simulink model "power_PSS_modif"  (R2021b)
settings: Solver=ode23tb  StartTime=0.0  StopTime=20  MaxStep=1/60  RelTol=1e-3  EnableMultiTasking=on
undefined symbols (not defined in the file or in its folder): D1, Delta
libraries: spsThreePhaseFaultLib x11, spsGenericPowerSystemStabilizerLib x8, spsThreePhaseBreakerLib x6, spsThreePhaseParallelRLCLoadLib x6, spsLoadFlowBusLib x6, spsThreePhasePISectionLineLib x4, spsSynchronousMachinepuStandardLib x4, cstblocks x4, spsExcitationSystemLib x4, spsMultiBandPowerSystemStabilizerLib x4, spsSteamTurbineandGovernorLib x4, spsThreePhaseTransformerTwoWindingsLib x4
(part 1 of 2)
settings Model: FPTRunName=Active  Creator=The MathWorks, Inc.  LastModifiedBy=Pavel
settings SolverCC: ConsecutiveZCsStepRelTol=10*128*eps/2  AlgebraicLoopSolver=TrustRegion
settings DataIOCC: SaveFormat=Array  SaveOutput=off  SaveTime=off  ReturnWorkspaceOutputs=off  TimeSaveName=t  SignalLoggingName=sigsOut
settings OptimizationCC: BlockReduction=off  BooleanDataType=off  ExpressionDepthLimit=2147483647  InitFltsAndDblsToZero=on  LifeSpan=inf
settings DebuggingCC: UnderspecifiedInitializationDetection=Classic  MergeDetectMultiDrivingBlocksExec=none  SignalResolutionControl=TryResolveAllWithWarning  MultiTaskDSMMsg=warning  MultiTaskCondExecSysMsg=none  FcnCallInpInsideContextMsg=warning  UnconnectedInputMsg=none  UnconnectedOutputMsg=none  UnconnectedLineMsg=none  StateNameClashWarn=warning  SFUnexpectedBacktrackingDiag=warning  SFNoUnconditionalDefaultTransitionDiag=warning  SFExecutionAtInitializationDiag=none  SFMachineParentedDataDiag=warning  ArithmeticOperatorsInVariantConditions=warning
settings HardwareCC: ProdBitPerPointer=32  ProdBitPerSizeT=32  ProdBitPerPtrDiffT=32  ProdLargestAtomicFloat=None  ProdIntDivRoundTo=Undefined  ProdEndianess=Unspecified  ProdWordSize=32  ProdHWDeviceType=32-bit Generic  TargetUnknown=on
settings ModelReferenceCC: PropagateSignalLabelsOutOfModel=off
settings SFSimCC: SimUseLocalCustomCode=off  CustomCodeUndefinedFunction=UseInterfaceOnly
settings RTWCC: RTWUseLocalCustomCode=off
settings CodeAppCC: StateflowObjectComments=on
settings GRTTargetCC: TargetLangStandard=C89/C90 (ANSI)  CombineOutputUpdateFcns=off  GRTInterface=on
settings ConfigComp: CovMetricSettings=dw  CovSaveCumulativeToWorkspaceVar=on  CovSaveSingleToWorkspaceVar=on  CovExternalEMLEnable=off  CovSFcnEnable=off
settings SimscapeCC: SimscapeNormalizeSystem=off

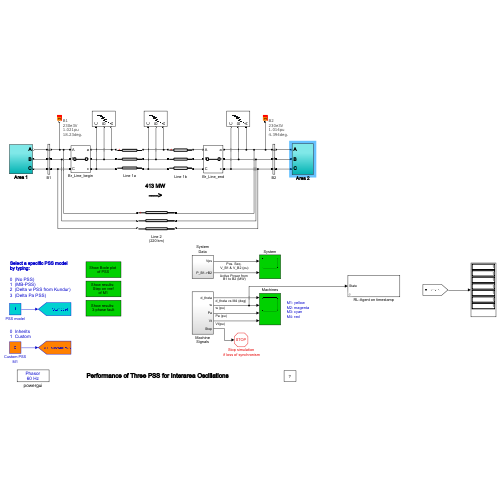
[thumbnail: Simulink's stored preview of the top-level diagram]
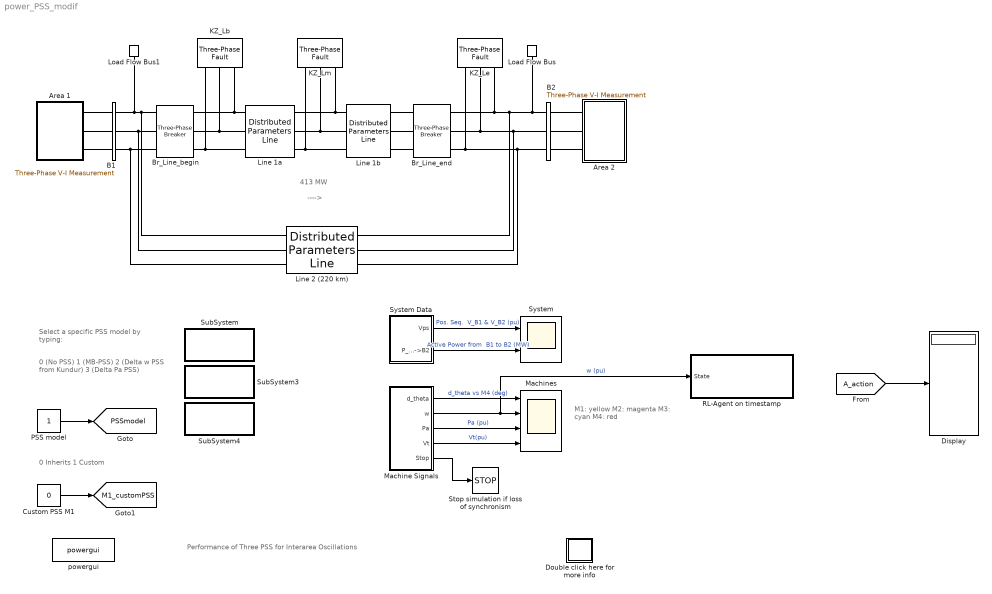
== system power_PSS_modif ==
  note: Performance of Three PSS for Interarea Oscillations
  note: M1: yellow
      | M2: magenta
      | M3: cyan
      | M4: red
  note: ---->
  note: 413 MW
  note: Select a specific PSS model
      | by typing:
  note: 0  (No PSS)
      | 1  (MB-PSS)
      | 2  (Delta w PSS from Kundur)
      | 3  (Delta Pa PSS)
  note: 0  Inherits
      | 1  Custom
  Area 1 : Subsystem
  Area 2 : Subsystem
  B1 : spsThreePhaseVIMeasurementLib/Three-Phase V-I Measurement  VoltageMeasurement=phase-to-ground  SetLabelV=on  LabelV=Vabc_B1  Vpu=off  VpuLL=off  CurrentMeasurement=yes  SetLabelI=on  LabelI=Iabc_B1  Ipu=off  Pbase=100e6  Vbase=500e3  OutputType=Complex  PhasorSimulation=on  PSBequivalent=0
  B2 : spsThreePhaseVIMeasurementLib/Three-Phase V-I Measurement  VoltageMeasurement=phase-to-ground  SetLabelV=on  LabelV=Vabc_B2  Vpu=off  VpuLL=off  CurrentMeasurement=yes  SetLabelI=on  LabelI=Iabc_B2  Ipu=off  Pbase=100e6  Vbase=500e3  OutputType=Complex  PhasorSimulation=on  PSBequivalent=0
  Br_Line_begin : spsThreePhaseBreakerLib/Three-Phase Breaker  InitialState=closed  SwitchA=on  SwitchB=on  SwitchC=on  SwitchTimes=[200]  External=off  BreakerResistance=0.001  SnubberResistance=inf  SnubberCapacitance=0  Measurements=None
      settings: AttributesFormatString=\n
  Br_Line_end : spsThreePhaseBreakerLib/Three-Phase Breaker  InitialState=closed  SwitchA=on  SwitchB=on  SwitchC=on  SwitchTimes=[200]  External=off  BreakerResistance=0.001  SnubberResistance=1e6  SnubberCapacitance=0  Measurements=None
      settings: AttributesFormatString=\n
  Custom PSS M1 : Constant  Value=0
  Display : Display
  Double click here for more info : Subsystem
      settings: OpenFcn=showdemo(bdroot(gcb))
      mask Display: disp('?')
  KZ_Lb : spsThreePhaseFaultLib/Three-Phase Fault  InitialStates=0  FaultA=off  FaultB=off  FaultC=off  GroundFault=on  SwitchTimes=[200]  External=off  SwitchStatus=NaN  FaultResistance=0.001  GroundResistance=0.001  SnubberResistance=1e6  SnubberCapacitance=inf  Measurements=None
  KZ_Le : spsThreePhaseFaultLib/Three-Phase Fault  InitialStates=0  FaultA=off  FaultB=off  FaultC=off  GroundFault=on  SwitchTimes=[200]  External=off  SwitchStatus=NaN  FaultResistance=0.001  GroundResistance=0.001  SnubberResistance=1e6  SnubberCapacitance=inf  Measurements=None
  KZ_Lm : spsThreePhaseFaultLib/Three-Phase Fault  InitialStates=0  FaultA=off  FaultB=off  FaultC=off  GroundFault=on  SwitchTimes=[200]  External=off  SwitchStatus=NaN  FaultResistance=0.001  GroundResistance=0.001  SnubberResistance=1e6  SnubberCapacitance=inf  Measurements=None
  Line 1a : spsDistributedParametersLineLib/Distributed Parameters Line  Phases=3  Length=110  Frequency=60  Resistance=[0.0529 1.61]  Inductance=[0.0014 0.0061]  Capacitance=[8.7749e-09 5.2489e-9]  x1=[1.03773522276635e-06 234865.712999227 234865.053199663;376.991118430775 376.991118430775 376.991118430775;-1.21492962029648 0.696371249684053 -0.874426885252841]  x2=[3.61832872068075e-07 234843.084420295 234843.00158467;376.991118430775 376.991118430775 376.991118430775;-0.99576107962275 0.574972704815849 -0.995825577248911]  x3=[1.73199030756503e-09 113.250290763104 113.254587804603;376.991118430775 376.991118430775 376.991118430775;0.426743142743769 0.12796103659155 -1.44291411331487]  x4=[2.20712280626888e-09 1062.45863712437 1062.45699915125;376.991118430775 376.991118430775 376.991118430775;-2.17151775162568 0.607648358429257 -0.963140711345587]  x5=0.000622431770558027  V1=ones(3,3)  V2=ones(3,3)  I1=ones(3,3)  I2=ones(3,3)  nHarmo=1  Measurements=None  Decoupling=off  VsMag0=0  VrMag0=0  VsAngle0=0  VrAngle0=0  IsMag0=0  IrMag0=0  IsAngle0=0  IrAngle0=0
      settings: AttributesFormatString=\n  SourceProductBaseCode=PS
  Line 1b : spsDistributedParametersLineLib/Distributed Parameters Line  Phases=3  Length=110  Frequency=60  Resistance=[0.0529 1.61]  Inductance=[0.0014 0.0061]  Capacitance=[8.7749e-09 5.2489e-9]  x1=[3.61827603793127e-07 234843.084420295 234843.00158467;376.991118430775 376.991118430775 376.991118430775;-0.995774949247956 0.574972704815849 -0.995825577248911]  x2=[3.91159002907788e-07 233276.177129905 233276.6633314;376.991118430775 376.991118430775 376.991118430775;1.48599709564018 0.454941358463387 -1.11585647609775]  x3=[2.05241143482151e-09 107.229638862451 107.234251771631;376.991118430775 376.991118430775 376.991118430775;0.699241722974643 0.245334104052737 -1.32554535066755]  x4=[1.87375449005804e-09 1055.26028297532 1055.25866903581;376.991118430775 376.991118430775 376.991118430775;-2.39378343032615 0.462097686461629 -1.10869145435477]  x5=0.000622431770558027  V1=ones(3,3)  V2=ones(3,3)  I1=ones(3,3)  I2=ones(3,3)  nHarmo=1  Measurements=None  Decoupling=off  VsMag0=0  VrMag0=0  VsAngle0=0  VrAngle0=0  IsMag0=0  IrMag0=0  IsAngle0=0  IrAngle0=0
      settings: AttributesFormatString=\n  SourceProductBaseCode=PS
  Line 2 (220 km) : spsDistributedParametersLineLib/Distributed Parameters Line  Phases=3  Length=220  Frequency=60  Resistance=[0.0001*529 1.61]  Inductance=[0.001*529/(377) 0.0061]  Capacitance=[0.00175/529/(377) 5.2489e-9]  x1=[1.03587220395795e-06 234866.202959166 234865.543159038;376.991118430775 376.991118430775 376.991118430775;-1.45669181718141 0.550693672846279 -1.02010446204846]  x2=[3.84671171209545e-07 233275.696082472 233276.182286874;376.991118430775 376.991118430775 376.991118430775;1.25538564201445 0.309263487558995 -1.26153434704163]  x3=[1.59106685653725e-09 111.016553993005 111.020863873188;376.991118430775 376.991118430775 376.991118430775;0.203367965270843 -0.0239956419974053 -1.59487136078097]  x4=[1.73228997364306e-09 1043.99344327446 1043.99184261649;376.991118430775 376.991118430775 376.991118430775;-2.6313512786114 0.316034427449977 -1.25475470203141]  x5=0.00124486354111605  V1=ones(3,3)  V2=ones(3,3)  I1=ones(3,3)  I2=ones(3,3)  nHarmo=1  Measurements=None  Decoupling=off  VsMag0=0  VrMag0=0  VsAngle0=0  VrAngle0=0  IsMag0=0  IrMag0=0  IsAngle0=0  IrAngle0=0
      settings: AttributesFormatString=\n  SourceProductBaseCode=PS
  Load Flow Bus : spsLoadFlowBusLib/Load Flow Bus  LConnTagsString=a  Phases=single  Connectors=on one side  ID=B2  Vbase=230e3  Vref=1  Vangle=0  VLF=1.014  VLFb=1  VLFc=1  angleLF=4.394  angleLFb=0  angleLFc=0
      settings: AttributesFormatString=%<ID>\n%<Vbase>V\n%<VLF>pu\n%<angleLF>deg.  SourceProductBaseCode=PS
  Load Flow Bus1 : spsLoadFlowBusLib/Load Flow Bus  LConnTagsString=a  Phases=single  Connectors=on one side  ID=B1  Vbase=230e3  Vref=1  Vangle=0  VLF=1.021  VLFb=1  VLFc=1  angleLF=18.23  angleLFb=0  angleLFc=0
      settings: AttributesFormatString=%<ID>\n%<Vbase>V\n%<VLF>pu\n%<angleLF>deg.  SourceProductBaseCode=PS
  Machine Signals : Subsystem
  Machines : Scope  NumInputPorts=4
  PSS model : Constant
  RL-Agent on timestamp : Subsystem  mask{period=1, swi_threshlod=1.1, initPSSParams=[1 1 1 1 1 1 1]}
      mask prompts: period "Period (s)"; swi_threshlod "Switch threshold (s)"; initPSSParams "Initial PSS parameters"
  Stop simulation if loss of synchronism : Stop
  SubSystem : Subsystem
      settings: OpenFcn=openfig('psbPSSbode.fig');
      mask Display: disp('Show Bode plot \nof PSS')
  SubSystem3 : Subsystem
      settings: OpenFcn=openfig('psbPSSstep.fig');
      mask Display: disp('Show results: \nStep on vref\nof M1')
  SubSystem4 : Subsystem
      settings: OpenFcn=openfig('psbPSSfault.fig');
      mask Display: disp('Show results: \n3-phase fault')
  System : Scope  NumInputPorts=2
  System Data : Subsystem
  powergui : spspowerguiLib/powergui  Priority=2  SimulationMode=Phasor  SampleTime=0  frequency=60  Iterations=50  frequencyindice=60  Pbase=100e6  ErrMax=0.0001  UnitsV=kV  UnitsW=MW  buscounter=0  FunctionMessages=off  echomessages=off  EnableUseOfTLC=off  CurrentSourceSwitches=off  DisableSnubberDevices=off  DisableRonSwitches=off  DisableVfSwitches=off  DisplayEquations=off  AutomaticDiscreteSolvers=off  SolverType=Tustin  Interpol=off  ExternalGateDelay=off  methode=off  Ts=0  x0status=blocks  SPID=off  SwTol=0  HookPort=off  NonlinearTolerance=1e-4  nMaxIteration=100  ContinueOnMaxIteration=off  RestoreLinks=warning  ResistiveCurrentMeasurement=off  Frange=logspace(0,3,50)  Ylog=off  Xlog=off  ShowGrid=off  save=off  variable=ZData  structure=0  ZoomFFT=on  StartTime=0.0  cycles=1  DisplayStyle=1  fundamental=60  FreqAxis=off  MaxFrequency=1000  frequencyindicesteady=1  RmsSteady=1  display=off
  tag scope: M1_customPSS=global, PSSmodel=global
  wires:
  Machine Signals/1(d_theta) -> Machines/1  "d_theta vs M4 (deg)"
  Machine Signals/2(w) -> RL-Agent on timestamp/1(State), Machines/2  "w (pu)"
  Machine Signals/3(Pa) -> Machines/3  "Pa (pu)"
  Machine Signals/4(Vt) -> Machines/4  "Vt(pu)"
  Machine Signals/5(Stop) -> Stop simulation if loss of synchronism/1
  System Data/1(Vps) -> System/1  "Pos. Seq.  V_B1 & V_B2 (pu)"
  System Data/2(P_B1->B2) -> System/2  "Active Power from  B1 to B2 (MW)"
  PSS model/1 -> [PSSmodel]
  [A_action] -> Display/1
  Custom PSS M1/1 -> [M1_customPSS]
  connections:
  Br_Line_begin/RConn1 -- KZ_Lb/LConn1 -- Line 1a/LConn1
  Br_Line_begin/RConn2 -- KZ_Lb/LConn2 -- Line 1a/LConn2
  Br_Line_begin/RConn3 -- KZ_Lb/LConn3 -- Line 1a/LConn3
  Line 1b/LConn1 -- KZ_Lm/LConn1 -- Line 1a/RConn1
  Line 1b/LConn2 -- KZ_Lm/LConn2 -- Line 1a/RConn2
  Line 1a/RConn3 -- KZ_Lm/LConn3 -- Line 1b/LConn3
  Line 1b/RConn1 -- Br_Line_end/LConn1
  Line 1b/RConn2 -- Br_Line_end/LConn2
  Line 1b/RConn3 -- Br_Line_end/LConn3
  Area 1/RConn2 -- B1/LConn2
  Area 1/RConn1 -- B1/LConn1
  Area 1/RConn3 -- B1/LConn3
  B1/RConn2 -- Br_Line_begin/LConn2 -- Line 2 (220 km)/LConn2
  B1/RConn1 -- Br_Line_begin/LConn1 -- Line 2 (220 km)/LConn1 -- Load Flow Bus1/LConn1
  B1/RConn3 -- Br_Line_begin/LConn3 -- Line 2 (220 km)/LConn3
  B2/RConn2 -- Area 2/LConn2
  B2/RConn1 -- Area 2/LConn1
  B2/RConn3 -- Area 2/LConn3
  B2/LConn2 -- KZ_Le/LConn2 -- Br_Line_end/RConn2 -- Line 2 (220 km)/RConn2
  B2/LConn1 -- KZ_Le/LConn1 -- Br_Line_end/RConn1 -- Line 2 (220 km)/RConn1 -- Load Flow Bus/LConn1
  B2/LConn3 -- KZ_Le/LConn3 -- Br_Line_end/RConn3 -- Line 2 (220 km)/RConn3

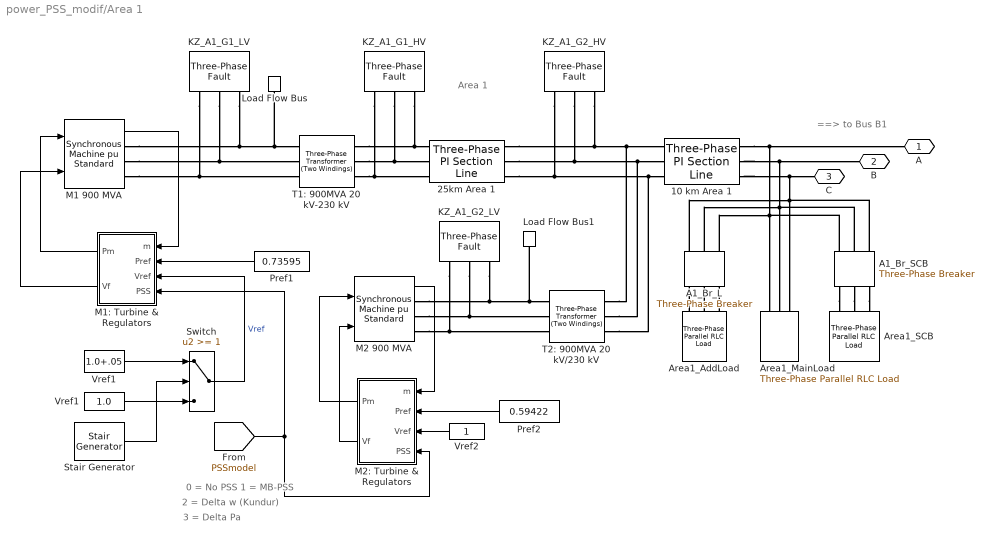
== system power_PSS_modif/Area 1 ==
  note: Area 1
  note: ==> to Bus B1
  note: 0 = No PSS
      | 1 = MB-PSS
  note: 3 = Delta Pa
  note: 2 = Delta w (Kundur)
  10 km Area 1 : spsThreePhasePISectionLineLib/Three-Phase PI Section Line  LConnTagsString=a|b|c  RConnTagsString=A|B|C  Length=10  Frequency=60  Resistances=[0.0529 1.61]  Inductances=[0.0014 0.0061]  Capacitances=[8.7749e-09 5.2489e-9]
  25km Area 1 : spsThreePhasePISectionLineLib/Three-Phase PI Section Line  LConnTagsString=a|b|c  RConnTagsString=A|B|C  Length=25  Frequency=60  Resistances=[0.0529 1.61]  Inductances=[0.0014 0.0061]  Capacitances=[8.7749e-09 5.2489e-9]
  A1_Br_L : spsThreePhaseBreakerLib/Three-Phase Breaker  InitialState=open  SwitchA=on  SwitchB=on  SwitchC=on  SwitchTimes=[200]  External=off  BreakerResistance=0.001  SnubberResistance=inf  SnubberCapacitance=0  Measurements=None
      settings: AttributesFormatString=\n
  A1_Br_SCB : spsThreePhaseBreakerLib/Three-Phase Breaker  InitialState=closed  SwitchA=on  SwitchB=on  SwitchC=on  SwitchTimes=[200]  External=off  BreakerResistance=0.001  SnubberResistance=inf  SnubberCapacitance=0  Measurements=None
      settings: AttributesFormatString=\n
  Area1_AddLoad : spsThreePhaseParallelRLCLoadLib/Three-Phase Parallel RLC Load  LConnTagsString=A|B|C  Configuration=Y (grounded)  NominalVoltage=230e3  Vabc=[1e3 1e3 1e3]  Vabcp=[1e3 1e3 1e3]  NominalFrequency=60  UnbalancedPower=off  ActivePower=1  InductivePower=0  CapacitivePower=0  Pabc=[10e3 9e3 11e3]  QLabc=[100 90 110]  QCabc=[100 90 110]  Pabcp=[10e3 9e3 11e3]  QLabcp=[100 90 110]  QCabcp=[100 90 110]  Measurements=None  LoadType=constant Z
  Area1_MainLoad : spsThreePhaseParallelRLCLoadLib/Three-Phase Parallel RLC Load  LConnTagsString=A|B|C  Configuration=Y (grounded)  NominalVoltage=230e3  Vabc=[1e3 1e3 1e3]  Vabcp=[1e3 1e3 1e3]  NominalFrequency=60  UnbalancedPower=off  ActivePower=900000000  InductivePower=0  CapacitivePower=100000000  Pabc=[10e3 9e3 11e3]  QLabc=[100 90 110]  QCabc=[100 90 110]  Pabcp=[10e3 9e3 11e3]  QLabcp=[100 90 110]  QCabcp=[100 90 110]  Measurements=None  LoadType=constant Z
  Area1_SCB : spsThreePhaseParallelRLCLoadLib/Three-Phase Parallel RLC Load  LConnTagsString=A|B|C  Configuration=Y (grounded)  NominalVoltage=230e3  Vabc=[1e3 1e3 1e3]  Vabcp=[1e3 1e3 1e3]  NominalFrequency=60  UnbalancedPower=off  ActivePower=0  InductivePower=0  CapacitivePower=200000000  Pabc=[10e3 9e3 11e3]  QLabc=[100 90 110]  QCabc=[100 90 110]  Pabcp=[10e3 9e3 11e3]  QLabcp=[100 90 110]  QCabcp=[100 90 110]  Measurements=None  LoadType=constant Z
  KZ_A1_G1_HV : spsThreePhaseFaultLib/Three-Phase Fault  InitialStates=0  FaultA=off  FaultB=off  FaultC=off  GroundFault=on  SwitchTimes=[200]  External=off  SwitchStatus=NaN  FaultResistance=0.001  GroundResistance=0.001  SnubberResistance=1e6  SnubberCapacitance=inf  Measurements=None
  KZ_A1_G1_LV : spsThreePhaseFaultLib/Three-Phase Fault  InitialStates=0  FaultA=off  FaultB=off  FaultC=off  GroundFault=on  SwitchTimes=[200]  External=off  SwitchStatus=NaN  FaultResistance=0.001  GroundResistance=0.001  SnubberResistance=1e6  SnubberCapacitance=inf  Measurements=None
  KZ_A1_G2_HV : spsThreePhaseFaultLib/Three-Phase Fault  InitialStates=0  FaultA=on  FaultB=on  FaultC=on  GroundFault=on  SwitchTimes=[200]  External=off  SwitchStatus=NaN  FaultResistance=0.001  GroundResistance=0.001  SnubberResistance=1e6  SnubberCapacitance=inf  Measurements=None
  KZ_A1_G2_LV : spsThreePhaseFaultLib/Three-Phase Fault  InitialStates=0  FaultA=off  FaultB=off  FaultC=off  GroundFault=on  SwitchTimes=[200]  External=off  SwitchStatus=NaN  FaultResistance=0.001  GroundResistance=0.001  SnubberResistance=1e6  SnubberCapacitance=inf  Measurements=None
  Load Flow Bus : spsLoadFlowBusLib/Load Flow Bus  LConnTagsString=a  Phases=single  Connectors=on one side  ID=M1_Area1  Vbase=20e3  Vref=1  Vangle=0  VLF=1  VLFb=1  VLFc=1  angleLF=10.73  angleLFb=0  angleLFc=0
      settings: AttributesFormatString=%<ID>\n%<Vbase>V\n%<VLF>pu\n%<angleLF>deg.  SourceProductBaseCode=PS
  Load Flow Bus1 : spsLoadFlowBusLib/Load Flow Bus  LConnTagsString=a  Phases=single  Connectors=on one side  ID=M2_Area1  Vbase=20e3  Vref=1  Vangle=0  VLF=1  VLFb=1  VLFc=1  angleLF=0  angleLFb=0  angleLFc=0
      settings: AttributesFormatString=%<ID>\n%<Vbase>V\n%<VLF>pu\n%<angleLF>deg.  SourceProductBaseCode=PS
  M1 900 MVA : spsSynchronousMachinepuStandardLib/Synchronous Machine pu Standard  PresetModel=No  MechanicalLoad=Mechanical power Pm  ShowDetailedParameters=on  RotorType=Round  Units=per unit standard parameters  MeasurementBus=off  NominalParameters="[900E6  20000   60 ]"  Reactances1=[1.8 .3 .25 1.7 .55 .25 .2]  Reactances2=[ 1.305, 0.296, 0.252, 0.474, 0.243, 0.18 ]  dAxisTimeConstants=Open-circuit  qAxisTimeConstants=Open-circuit  TimeConstants1=[]  TimeConstants2=[8 .03 .4 .05]  TimeConstants3=[]  TimeConstants4=[]  TimeConstants5=[ 1.01, 0.053, 0.1 ]  TimeConstants6=[]  TimeConstants7=[]  TimeConstants8=[]  StatorResistance=0.0025  Mechanical=[ 6.5 0 4]  PolePairs=4  InitialConditions=[0 -29.8925 0.737138 0.737138 0.737138 7.47241 -112.528 127.472 1.70671]  SetSaturation=off  Saturation=[0.6404,0.7127,0.8441,0.9214,0.9956,1.082,1.19,1.316,1.457;0.7,0.7698,0.8872,0.9466,0.9969,1.046,1.1,1.151,1.201]  LoadFlowParameters=[1 700000000 0 0 0]  TsPowergui=0  TsBlock=-1  IterativeModel=Trapezoidal non iterative  IterativeDiscreteModel=Trapezoidal non iterative  BusType=PV  Pref=662353696.8626  Qref=0  Qmin=-Inf  Qmax=Inf  PLF=0  QLF=0
      settings: SourceProductBaseCode=PS
  M1: Turbine & Regulators : Subsystem
  M2 900 MVA : spsSynchronousMachinepuStandardLib/Synchronous Machine pu Standard  PresetModel=No  MechanicalLoad=Mechanical power Pm  ShowDetailedParameters=on  RotorType=Round  Units=per unit standard parameters  MeasurementBus=off  NominalParameters="[900E6  20000   60 ]"  Reactances1=[1.8 .3 .25 1.7 .55 .25 .2]  Reactances2=[ 1.305, 0.296, 0.252, 0.474, 0.243, 0.18 ]  dAxisTimeConstants=Open-circuit  qAxisTimeConstants=Open-circuit  TimeConstants1=[]  TimeConstants2=[8 .03 .4 .05]  TimeConstants3=[]  TimeConstants4=[]  TimeConstants5=[ 1.01, 0.053, 0.1 ]  TimeConstants6=[]  TimeConstants7=[]  TimeConstants8=[]  StatorResistance=0.0025  Mechanical=[ 6.5 0 4]  PolePairs=4  InitialConditions=[0 -44.1681 0.594337 0.594337 0.594337 1.14574 -118.854 121.146 1.45014]  SetSaturation=off  Saturation=[0.6404,0.7127,0.8441,0.9214,0.9956,1.082,1.19,1.316,1.457;0.7,0.7698,0.8872,0.9466,0.9969,1.046,1.1,1.151,1.201]  LoadFlowParameters=[2 700000000 0 0 0]  TsPowergui=0  TsBlock=-1  IterativeModel=Trapezoidal non iterative  IterativeDiscreteModel=Trapezoidal non iterative  BusType=swing  Pref=754208614.3715  Qref=0  Qmin=-Inf  Qmax=Inf  PLF=0  QLF=0
      settings: SourceProductBaseCode=PS
  M2: Turbine & Regulators : Subsystem
  Pref1 : Constant  Value=0.73595
  Pref2 : Constant  Value=0.59422
  Stair Generator : spsStairGeneratorLib/Stair Generator  t=[0 1 1.2]*100  e=[0 1 0 ]  Ts=0
  Switch : Switch  Threshold=1  InputSameDT=on
  T1: 900MVA 20 kV-230 kV : spsThreePhaseTransformerTwoWindingsLib/Three-Phase Transformer (Two Windings)  Winding1Connection=Delta (D1)  Winding2Connection=Yg  CoreType=Three single-phase transformers  SetSaturation=off  Hysteresis=off  DataFile='hysteresis'  SetInitialFlux=off  Measurements=None  UNITS=pu  NominalPower="[ 900e6   60 ]"  Winding1="[ 20e3  1e-6   0  ]"  Winding2="[ 230e3  1e-6   0.15 ]"  Rm=500  Lm=500  L0=0.5  Saturation="[ 0,0  ;  0.005,1.2  ;  1.0,1.4 ]"  InitialFluxes=[ 0.8 , -0.8 , 0.7 ]  BreakLoop=off  DiscreteSolver=Trapezoidal iterative  DataType=off  TransfoNumber=0
  T2: 900MVA 20 kV/230 kV : spsThreePhaseTransformerTwoWindingsLib/Three-Phase Transformer (Two Windings)  Winding1Connection=Delta (D1)  Winding2Connection=Yg  CoreType=Three single-phase transformers  SetSaturation=off  Hysteresis=off  DataFile='hysteresis'  SetInitialFlux=off  Measurements=None  UNITS=pu  NominalPower=[ 900e6 60 ]  Winding1="[ 20e3 1e-6  0.0]"  Winding2=[ 230e3 1e-6 0.15]  Rm=500  Lm=500  L0=0.5  Saturation="[ 0,0  ;  0.005,1.2  ;  1.0,1.4 ]"  InitialFluxes=[ 0.8 , -0.8 , 0.7 ]  BreakLoop=off  DiscreteSolver=Trapezoidal iterative  DataType=off  TransfoNumber=0
  Vref1 : Constant  Value=1.0
  "Vref1 " : Constant  Value=1.0+.05
  Vref2 : Constant
  " A" : PMIOPort  Side=Right
  " B" : PMIOPort  Port=2  Side=Right
  " C" : PMIOPort  Port=3  Side=Right
  wires:
  Pref1/1 -> M1: Turbine & Regulators/2(Pref)
  Switch/1 -> M1: Turbine & Regulators/3(Vref)  "Vref"
  Stair Generator/1 -> Switch/2
  [PSSmodel] -> M1: Turbine & Regulators/4(PSS), M2: Turbine & Regulators/4(PSS)
  Pref2/1 -> M2: Turbine & Regulators/2(Pref)
  Vref2/1 -> M2: Turbine & Regulators/3(Vref)
  Vref1/1 -> Switch/3
  "Vref1 "/1 -> Switch/1
  M2 900 MVA/1 -> M2: Turbine & Regulators/1(m)
  M2: Turbine & Regulators/1(Pm) -> M2 900 MVA/1
  M2: Turbine & Regulators/2(Vf) -> M2 900 MVA/2
  M1: Turbine & Regulators/1(Pm) -> M1 900 MVA/1
  M1: Turbine & Regulators/2(Vf) -> M1 900 MVA/2
  M1 900 MVA/1 -> M1: Turbine & Regulators/1(m)
  connections:
  T1: 900MVA 20 kV-230 kV/RConn1 -- KZ_A1_G1_HV/LConn1 -- 25km Area 1/LConn1
  T1: 900MVA 20 kV-230 kV/RConn2 -- KZ_A1_G1_HV/LConn2 -- 25km Area 1/LConn2
  M2 900 MVA/RConn1 -- KZ_A1_G2_LV/LConn1 -- T2: 900MVA 20 kV/230 kV/LConn1 -- Load Flow Bus1/LConn1
  M2 900 MVA/RConn2 -- KZ_A1_G2_LV/LConn2 -- T2: 900MVA 20 kV/230 kV/LConn2
  M2 900 MVA/RConn3 -- KZ_A1_G2_LV/LConn3 -- T2: 900MVA 20 kV/230 kV/LConn3
  T1: 900MVA 20 kV-230 kV/RConn3 -- KZ_A1_G1_HV/LConn3 -- 25km Area 1/LConn3
  10 km Area 1/RConn1 -- " A"/RConn1 -- A1_Br_L/RConn3 -- A1_Br_SCB/RConn1 -- Area1_MainLoad/LConn1
  10 km Area 1/RConn2 -- " B"/RConn1 -- A1_Br_L/RConn2 -- A1_Br_SCB/RConn2 -- Area1_MainLoad/LConn2
  10 km Area 1/RConn3 -- " C"/RConn1 -- A1_Br_L/RConn1 -- A1_Br_SCB/RConn3 -- Area1_MainLoad/LConn3
  M1 900 MVA/RConn1 -- KZ_A1_G1_LV/LConn1 -- T1: 900MVA 20 kV-230 kV/LConn1 -- Load Flow Bus/LConn1
  M1 900 MVA/RConn2 -- KZ_A1_G1_LV/LConn2 -- T1: 900MVA 20 kV-230 kV/LConn2
  M1 900 MVA/RConn3 -- KZ_A1_G1_LV/LConn3 -- T1: 900MVA 20 kV-230 kV/LConn3
  25km Area 1/RConn2 -- KZ_A1_G2_HV/LConn2 -- T2: 900MVA 20 kV/230 kV/RConn2 -- 10 km Area 1/LConn2
  25km Area 1/RConn1 -- KZ_A1_G2_HV/LConn1 -- T2: 900MVA 20 kV/230 kV/RConn1 -- 10 km Area 1/LConn1
  25km Area 1/RConn3 -- KZ_A1_G2_HV/LConn3 -- T2: 900MVA 20 kV/230 kV/RConn3 -- 10 km Area 1/LConn3
  A1_Br_SCB/LConn1 -- Area1_SCB/LConn1
  A1_Br_SCB/LConn2 -- Area1_SCB/LConn2
  A1_Br_SCB/LConn3 -- Area1_SCB/LConn3
  Area1_AddLoad/LConn1 -- A1_Br_L/LConn1
  Area1_AddLoad/LConn3 -- A1_Br_L/LConn3
  Area1_AddLoad/LConn2 -- A1_Br_L/LConn2

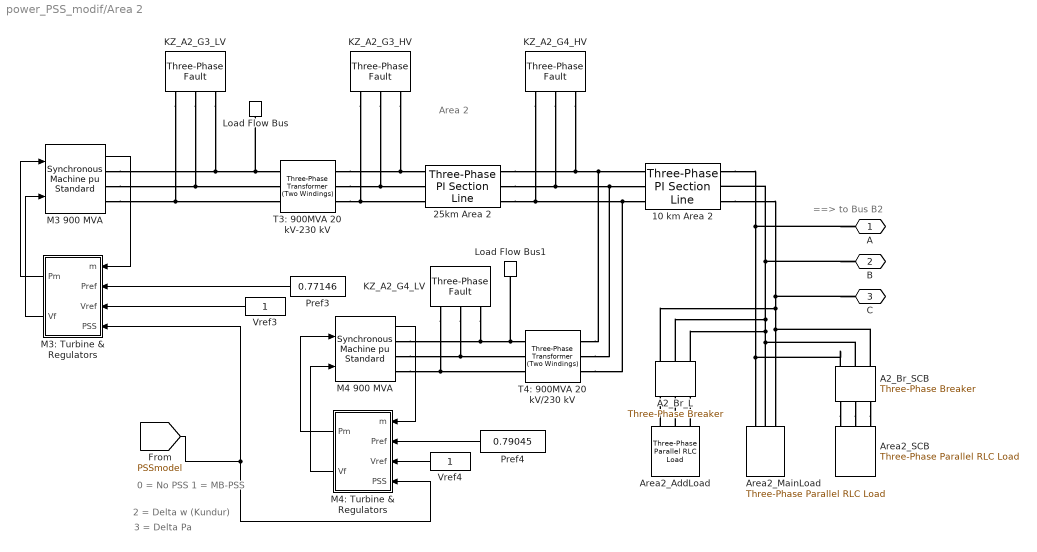
== system power_PSS_modif/Area 2 ==
  note: 2 = Delta w (Kundur)
  note: 3 = Delta Pa
  note: 0 = No PSS
      | 1 = MB-PSS
  note: ==> to Bus B2
  note: Area 2
  10 km Area 2 : spsThreePhasePISectionLineLib/Three-Phase PI Section Line  LConnTagsString=a|b|c  RConnTagsString=A|B|C  Length=10  Frequency=60  Resistances=[0.0529 1.61]  Inductances=[0.0014 0.0061]  Capacitances=[8.7749e-09 5.2489e-9]
  25km Area 2 : spsThreePhasePISectionLineLib/Three-Phase PI Section Line  LConnTagsString=a|b|c  RConnTagsString=A|B|C  Length=25  Frequency=60  Resistances=[0.0529 1.61]  Inductances=[0.0014 0.0061]  Capacitances=[8.7749e-09 5.2489e-9]
  A2_Br_L : spsThreePhaseBreakerLib/Three-Phase Breaker  InitialState=open  SwitchA=on  SwitchB=on  SwitchC=on  SwitchTimes=[200]  External=off  BreakerResistance=0.001  SnubberResistance=inf  SnubberCapacitance=0  Measurements=None
      settings: AttributesFormatString=\n
  A2_Br_SCB : spsThreePhaseBreakerLib/Three-Phase Breaker  InitialState=closed  SwitchA=on  SwitchB=on  SwitchC=on  SwitchTimes=[200]  External=off  BreakerResistance=0.001  SnubberResistance=inf  SnubberCapacitance=0  Measurements=None
      settings: AttributesFormatString=\n
  Area2_AddLoad : spsThreePhaseParallelRLCLoadLib/Three-Phase Parallel RLC Load  LConnTagsString=A|B|C  Configuration=Y (grounded)  NominalVoltage=230e3  Vabc=[1e3 1e3 1e3]  Vabcp=[1e3 1e3 1e3]  NominalFrequency=60  UnbalancedPower=off  ActivePower=200  InductivePower=0  CapacitivePower=1  Pabc=[10e3 9e3 11e3]  QLabc=[100 90 110]  QCabc=[100 90 110]  Pabcp=[10e3 9e3 11e3]  QLabcp=[100 90 110]  QCabcp=[100 90 110]  Measurements=None  LoadType=constant Z
  Area2_MainLoad : spsThreePhaseParallelRLCLoadLib/Three-Phase Parallel RLC Load  LConnTagsString=A|B|C  Configuration=Y (grounded)  NominalVoltage=230e3  Vabc=[1e3 1e3 1e3]  Vabcp=[1e3 1e3 1e3]  NominalFrequency=60  UnbalancedPower=off  ActivePower=1550000000  InductivePower=0  CapacitivePower=19684279.1507  Pabc=[10e3 9e3 11e3]  QLabc=[100 90 110]  QCabc=[100 90 110]  Pabcp=[10e3 9e3 11e3]  QLabcp=[100 90 110]  QCabcp=[100 90 110]  Measurements=None  LoadType=constant Z
  Area2_SCB : spsThreePhaseParallelRLCLoadLib/Three-Phase Parallel RLC Load  LConnTagsString=A|B|C  Configuration=Y (grounded)  NominalVoltage=230e3  Vabc=[1e3 1e3 1e3]  Vabcp=[1e3 1e3 1e3]  NominalFrequency=60  UnbalancedPower=off  ActivePower=0  InductivePower=0  CapacitivePower=350000000  Pabc=[10e3 9e3 11e3]  QLabc=[100 90 110]  QCabc=[100 90 110]  Pabcp=[10e3 9e3 11e3]  QLabcp=[100 90 110]  QCabcp=[100 90 110]  Measurements=None  LoadType=constant Z
  KZ_A2_G3_HV : spsThreePhaseFaultLib/Three-Phase Fault  InitialStates=0  FaultA=off  FaultB=off  FaultC=off  GroundFault=on  SwitchTimes=[200]  External=off  SwitchStatus=NaN  FaultResistance=0.001  GroundResistance=0.001  SnubberResistance=1e6  SnubberCapacitance=inf  Measurements=None
  KZ_A2_G3_LV : spsThreePhaseFaultLib/Three-Phase Fault  InitialStates=0  FaultA=off  FaultB=off  FaultC=off  GroundFault=on  SwitchTimes=[200]  External=off  SwitchStatus=NaN  FaultResistance=0.001  GroundResistance=0.001  SnubberResistance=1e6  SnubberCapacitance=inf  Measurements=None
  KZ_A2_G4_HV : spsThreePhaseFaultLib/Three-Phase Fault  InitialStates=0  FaultA=off  FaultB=off  FaultC=off  GroundFault=on  SwitchTimes=[200]  External=off  SwitchStatus=NaN  FaultResistance=0.001  GroundResistance=0.001  SnubberResistance=1e6  SnubberCapacitance=inf  Measurements=None
  KZ_A2_G4_LV : spsThreePhaseFaultLib/Three-Phase Fault  InitialStates=0  FaultA=off  FaultB=off  FaultC=off  GroundFault=on  SwitchTimes=[200]  External=off  SwitchStatus=NaN  FaultResistance=0.001  GroundResistance=0.001  SnubberResistance=1e6  SnubberCapacitance=inf  Measurements=None
  Load Flow Bus : spsLoadFlowBusLib/Load Flow Bus  LConnTagsString=a  Phases=single  Connectors=on one side  ID=M3_Area2  Vbase=20e3  Vref=1  Vangle=0  VLF=1  VLFb=1  VLFc=1  angleLF=-0.9983  angleLFb=0  angleLFc=0
      settings: AttributesFormatString=%<ID>\n%<Vbase>V\n%<VLF>pu\n%<angleLF>deg.  SourceProductBaseCode=PS
  Load Flow Bus1 : spsLoadFlowBusLib/Load Flow Bus  LConnTagsString=a  Phases=single  Connectors=on one side  ID=M4_Area2  Vbase=20e3  Vref=1  Vangle=0  VLF=1  VLFb=1  VLFc=1  angleLF=-10.86  angleLFb=0  angleLFc=0
      settings: AttributesFormatString=%<ID>\n%<Vbase>V\n%<VLF>pu\n%<angleLF>deg.  SourceProductBaseCode=PS
  M3 900 MVA : spsSynchronousMachinepuStandardLib/Synchronous Machine pu Standard  PresetModel=No  MechanicalLoad=Mechanical power Pm  ShowDetailedParameters=on  RotorType=Round  Units=per unit standard parameters  MeasurementBus=off  NominalParameters="[900E6  20000   60 ]"  Reactances1=[1.8 .3 .25 1.7 .55 .25 .2]  Reactances2=[ 1.305, 0.296, 0.252, 0.474, 0.243, 0.18 ]  dAxisTimeConstants=Open-circuit  qAxisTimeConstants=Open-circuit  TimeConstants1=[]  TimeConstants2=[8 .03 .4 .05]  TimeConstants3=[]  TimeConstants4=[]  TimeConstants5=[ 1.01, 0.053, 0.1 ]  TimeConstants6=[]  TimeConstants7=[]  TimeConstants8=[]  StatorResistance=0.0025  Mechanical=[ 6.175 0 4]  PolePairs=4  InitialConditions=[0 -41.3376 0.77425 0.77425 0.77425 -5.86613 -125.866 114.134 1.78343]  SetSaturation=off  Saturation=[0.6404,0.7127,0.8441,0.9214,0.9956,1.082,1.19,1.316,1.457;0.7,0.7698,0.8872,0.9466,0.9969,1.046,1.1,1.151,1.201]  LoadFlowParameters=[1 719000000 0 0 0]  TsPowergui=0  TsBlock=-1  IterativeModel=Trapezoidal non iterative  IterativeDiscreteModel=Trapezoidal non iterative  BusType=PV  Pref=694311768.0691  Qref=0  Qmin=-Inf  Qmax=Inf  PLF=0  QLF=0
      settings: SourceProductBaseCode=PS
  M3: Turbine & Regulators : Subsystem
  M4 900 MVA : spsSynchronousMachinepuStandardLib/Synchronous Machine pu Standard  PresetModel=No  MechanicalLoad=Mechanical power Pm  ShowDetailedParameters=on  RotorType=Round  Units=per unit standard parameters  MeasurementBus=off  NominalParameters="[900E6  20000   60 ]"  Reactances1=[1.8 .3 .25 1.7 .55 .25 .2]  Reactances2=[ 1.305, 0.296, 0.252, 0.474, 0.243, 0.18 ]  dAxisTimeConstants=Open-circuit  qAxisTimeConstants=Open-circuit  TimeConstants1=[]  TimeConstants2=[8 .03 .4 .05]  TimeConstants3=[]  TimeConstants4=[]  TimeConstants5=[ 1.01, 0.053, 0.1 ]  TimeConstants6=[]  TimeConstants7=[]  TimeConstants8=[]  StatorResistance=0.0025  Mechanical=[ 6.175 0 4]  PolePairs=4  InitialConditions=[0 -49.7051 0.791857 0.791857 0.791857 -14.2734 -134.273 105.727 1.7898]  SetSaturation=off  Saturation=[0.6404,0.7127,0.8441,0.9214,0.9956,1.082,1.19,1.316,1.457;0.7,0.7698,0.8872,0.9466,0.9969,1.046,1.1,1.151,1.201]  LoadFlowParameters=[1 700000000 0 0 0]  TsPowergui=0  TsBlock=-1  IterativeModel=Trapezoidal non iterative  IterativeDiscreteModel=Trapezoidal non iterative  BusType=PV  Pref=711403727.9223  Qref=0  Qmin=-Inf  Qmax=Inf  PLF=0  QLF=0
      settings: SourceProductBaseCode=PS
  M4: Turbine & Regulators : Subsystem
  Pref3 : Constant  Value=0.77146
  Pref4 : Constant  Value=0.79045
  T3: 900MVA 20 kV-230 kV : spsThreePhaseTransformerTwoWindingsLib/Three-Phase Transformer (Two Windings)  Winding1Connection=Delta (D1)  Winding2Connection=Yg  CoreType=Three single-phase transformers  SetSaturation=off  Hysteresis=off  DataFile='hysteresis'  SetInitialFlux=off  Measurements=None  UNITS=pu  NominalPower="[ 900e6   60 ]"  Winding1="[ 20e3  1e-6   0  ]"  Winding2="[ 230e3  1e-6   0.15 ]"  Rm=500  Lm=500  L0=0.5  Saturation="[ 0,0  ;  0.005,1.2  ;  1.0,1.4 ]"  InitialFluxes=[ 0.8 , -0.8 , 0.7 ]  BreakLoop=off  DiscreteSolver=Trapezoidal iterative  DataType=off  TransfoNumber=0
  T4: 900MVA 20 kV/230 kV : spsThreePhaseTransformerTwoWindingsLib/Three-Phase Transformer (Two Windings)  Winding1Connection=Delta (D1)  Winding2Connection=Yg  CoreType=Three single-phase transformers  SetSaturation=off  Hysteresis=off  DataFile='hysteresis'  SetInitialFlux=off  Measurements=None  UNITS=pu  NominalPower=[ 900e6 60 ]  Winding1="[ 20e3 1e-6  0.0]"  Winding2=[ 230e3 1e-6 0.15]  Rm=500  Lm=500  L0=0.5  Saturation="[ 0,0  ;  0.005,1.2  ;  1.0,1.4 ]"  InitialFluxes=[ 0.8 , -0.8 , 0.7 ]  BreakLoop=off  DiscreteSolver=Trapezoidal iterative  DataType=off  TransfoNumber=0
  Vref3 : Constant
  Vref4 : Constant
  A : PMIOPort  Side=Left
  B : PMIOPort  Port=2  Side=Left
  C : PMIOPort  Port=3  Side=Left
  wires:
  [PSSmodel] -> M3: Turbine & Regulators/4(PSS), M4: Turbine & Regulators/4(PSS)
  Pref3/1 -> M3: Turbine & Regulators/2(Pref)
  Vref3/1 -> M3: Turbine & Regulators/3(Vref)
  Pref4/1 -> M4: Turbine & Regulators/2(Pref)
  Vref4/1 -> M4: Turbine & Regulators/3(Vref)
  M3 900 MVA/1 -> M3: Turbine & Regulators/1(m)
  M3: Turbine & Regulators/2(Vf) -> M3 900 MVA/2
  M3: Turbine & Regulators/1(Pm) -> M3 900 MVA/1
  M4: Turbine & Regulators/1(Pm) -> M4 900 MVA/1
  M4: Turbine & Regulators/2(Vf) -> M4 900 MVA/2
  M4 900 MVA/1 -> M4: Turbine & Regulators/1(m)
  connections:
  M3 900 MVA/RConn3 -- KZ_A2_G3_LV/LConn3 -- T3: 900MVA 20 kV-230 kV/LConn3
  M3 900 MVA/RConn2 -- KZ_A2_G3_LV/LConn2 -- T3: 900MVA 20 kV-230 kV/LConn2
  M3 900 MVA/RConn1 -- KZ_A2_G3_LV/LConn1 -- T3: 900MVA 20 kV-230 kV/LConn1 -- Load Flow Bus/LConn1
  T3: 900MVA 20 kV-230 kV/RConn3 -- KZ_A2_G3_HV/LConn3 -- 25km Area 2/LConn3
  M4 900 MVA/RConn3 -- KZ_A2_G4_LV/LConn3 -- T4: 900MVA 20 kV/230 kV/LConn3
  M4 900 MVA/RConn2 -- KZ_A2_G4_LV/LConn2 -- T4: 900MVA 20 kV/230 kV/LConn2
  M4 900 MVA/RConn1 -- KZ_A2_G4_LV/LConn1 -- T4: 900MVA 20 kV/230 kV/LConn1 -- Load Flow Bus1/LConn1
  T3: 900MVA 20 kV-230 kV/RConn2 -- KZ_A2_G3_HV/LConn2 -- 25km Area 2/LConn2
  T3: 900MVA 20 kV-230 kV/RConn1 -- KZ_A2_G3_HV/LConn1 -- 25km Area 2/LConn1
  25km Area 2/RConn2 -- KZ_A2_G4_HV/LConn2 -- T4: 900MVA 20 kV/230 kV/RConn2 -- 10 km Area 2/LConn2
  25km Area 2/RConn1 -- KZ_A2_G4_HV/LConn1 -- T4: 900MVA 20 kV/230 kV/RConn1 -- 10 km Area 2/LConn1
  25km Area 2/RConn3 -- KZ_A2_G4_HV/LConn3 -- T4: 900MVA 20 kV/230 kV/RConn3 -- 10 km Area 2/LConn3
  10 km Area 2/RConn1 -- A2_Br_SCB/RConn1 -- Area2_MainLoad/LConn1 -- A/RConn1
  Area2_MainLoad/LConn2 -- A2_Br_SCB/RConn2 -- A2_Br_L/RConn3 -- A2_Br_L/RConn2 -- 10 km Area 2/RConn2 -- B/RConn1
  10 km Area 2/RConn3 -- A2_Br_L/RConn1 -- A2_Br_SCB/RConn3 -- Area2_MainLoad/LConn3 -- C/RConn1
  A2_Br_SCB/LConn1 -- Area2_SCB/LConn1
  A2_Br_SCB/LConn2 -- Area2_SCB/LConn2
  A2_Br_SCB/LConn3 -- Area2_SCB/LConn3
  Area2_AddLoad/LConn2 -- A2_Br_L/LConn2
  Area2_AddLoad/LConn3 -- A2_Br_L/LConn3
  Area2_AddLoad/LConn1 -- A2_Br_L/LConn1

== system power_PSS_modif/Double click here for more info ==

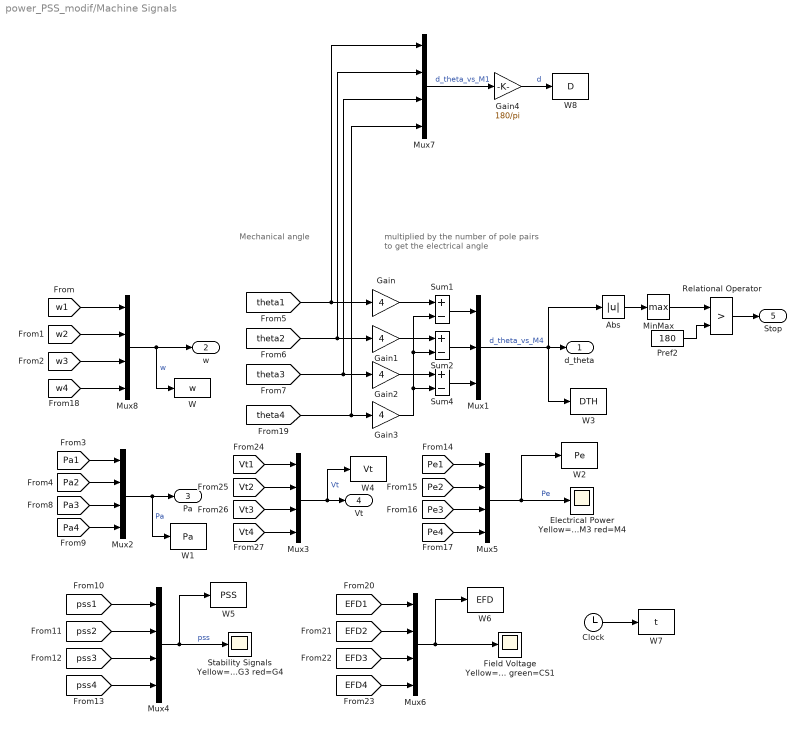
== system power_PSS_modif/Machine Signals ==
  note: Mechanical angle
  note: multiplied by the number of pole pairs
      | to get the electrical angle
  Abs : Abs  SaturateOnIntegerOverflow=on
  Clock : Clock
  "Electrical Power Yellow=M1 mag=M2 cyan=M3 red=M4 " : Scope
  Field Voltage Yellow=G1 mag=G2 cyan=G3 red=G4 green=CS1 : Scope
  Gain{,1..3} (4 alike) : Gain  Gain=4
  Gain4 : Gain  Gain=180/pi
  MinMax : MinMax  Function=max  InputSameDT=on  SaturateOnIntegerOverflow=on
  Mux1 : Mux  Inputs=3
  Mux{2..8} (7 alike) : Mux
  Pref2 : Constant  Value=180
  Relational Operator : RelationalOperator  Operator=>  RndMeth=Nearest  InputSameDT=on
  "Stability Signals Yellow=G1 mag=G2 cyan=G3 red=G4 " : Scope
  Sum1 : Sum  Inputs=+-  InputSameDT=on  SaturateOnIntegerOverflow=on  OutDataTypeStr=Inherit: Same as first input
  Sum2 : Sum  Inputs=+-  InputSameDT=on  SaturateOnIntegerOverflow=on  OutDataTypeStr=Inherit: Same as first input
  Sum4 : Sum  Inputs=+-  InputSameDT=on  SaturateOnIntegerOverflow=on  OutDataTypeStr=Inherit: Same as first input
  W : ToWorkspace  VariableName=w  SampleTime=1/60
  W1 : ToWorkspace  VariableName=Pa  SampleTime=1/60
  W2 : ToWorkspace  VariableName=Pe  SampleTime=1/60
  W3 : ToWorkspace  VariableName=DTH  SampleTime=1/60
  W4 : ToWorkspace  VariableName=Vt  SampleTime=1/60
  W5 : ToWorkspace  VariableName=PSS  SampleTime=1/60
  W6 : ToWorkspace  VariableName=EFD  SampleTime=1/60
  W7 : ToWorkspace  VariableName=t  SampleTime=1/60
  W8 : ToWorkspace  VariableName=D  SampleTime=-1
  d_theta : Outport  VectorParamsAs1DForOutWhenUnconnected=off
  w : Outport  Port=2  VectorParamsAs1DForOutWhenUnconnected=off
  Pa : Outport  Port=3  VectorParamsAs1DForOutWhenUnconnected=off
  Vt : Outport  Port=4  VectorParamsAs1DForOutWhenUnconnected=off
  Stop : Outport  Port=5  VectorParamsAs1DForOutWhenUnconnected=off
  wires:
  Mux1/1 -> d_theta/1, Abs/1, W3/1  "d_theta_vs_M4"
  Abs/1 -> MinMax/1
  Pref2/1 -> Relational Operator/2
  MinMax/1 -> Relational Operator/1
  [Pa1] -> Mux2/1
  Mux4/1 -> "Stability Signals Yellow=G1 mag=G2 cyan=G3 red=G4 "/1, W5/1  "pss"
  [pss1] -> Mux4/1
  [pss2] -> Mux4/2
  [pss4] -> Mux4/4
  [pss3] -> Mux4/3
  [EFD1] -> Mux6/1
  [EFD2] -> Mux6/2
  [EFD4] -> Mux6/4
  [EFD3] -> Mux6/3
  Mux6/1 -> Field Voltage Yellow=G1 mag=G2 cyan=G3 red=G4 green=CS1/1, W6/1
  Mux8/1 -> w/1, W/1  "w"
  Relational Operator/1 -> Stop/1
  Mux2/1 -> Pa/1, W1/1  "Pa"
  Sum1/1 -> Mux1/1
  Sum2/1 -> Mux1/2
  Sum4/1 -> Mux1/3
  [Pa2] -> Mux2/2
  [Pa3] -> Mux2/3
  [Pa4] -> Mux2/4
  [Vt1] -> Mux3/1
  [Vt2] -> Mux3/2
  [Vt3] -> Mux3/3
  [Vt4] -> Mux3/4
  Mux3/1 -> Vt/1, W4/1  "Vt"
  [Pe1] -> Mux5/1
  [Pe2] -> Mux5/2
  [Pe3] -> Mux5/3
  [Pe4] -> Mux5/4
  Mux5/1 -> "Electrical Power Yellow=M1 mag=M2 cyan=M3 red=M4 "/1, W2/1  "Pe"
  [w1] -> Mux8/1
  [w2] -> Mux8/2
  [w3] -> Mux8/3
  [w4] -> Mux8/4
  Clock/1 -> W7/1
  Gain/1 -> Sum1/1
  Gain1/1 -> Sum2/1
  Gain2/1 -> Sum4/1
  Gain3/1 -> Sum4/2, Sum2/2, Sum1/2
  [theta2] -> Mux7/2, Gain1/1
  [theta1] -> Mux7/1, Gain/1
  Gain4/1 -> W8/1  "d"
  [theta3] -> Mux7/3, Gain2/1
  Mux7/1 -> Gain4/1  "d_theta_vs_M1"
  [theta4] -> Mux7/4, Gain3/1

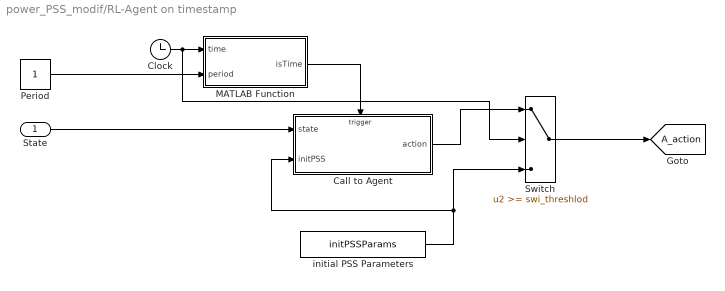
== system power_PSS_modif/RL-Agent on timestamp ==
  State : Inport
  Call to Agent : Subsystem
  Clock : Clock
  MATLAB Function : MATLAB Function  TreatAsAtomicUnit=on
  Period : Constant
  Switch : Switch  Threshold=swi_threshlod
  initial PSS Parameters : Constant  Value=initPSSParams  VectorParams1D=off
  tag scope: A_action=global
  wires:
  Clock/1 -> Switch/2, MATLAB Function/1(time)
  MATLAB Function/1(isTime) -> Call to Agent/Trigger
  State/1 -> Call to Agent/1(state)
  Period/1 -> MATLAB Function/2(period)
  Switch/1 -> [A_action]
  Call to Agent/1(action) -> Switch/1
  initial PSS Parameters/1 -> Switch/3, Call to Agent/2(initPSS)

== system power_PSS_modif/SubSystem ==

== system power_PSS_modif/SubSystem3 ==

== system power_PSS_modif/SubSystem4 ==

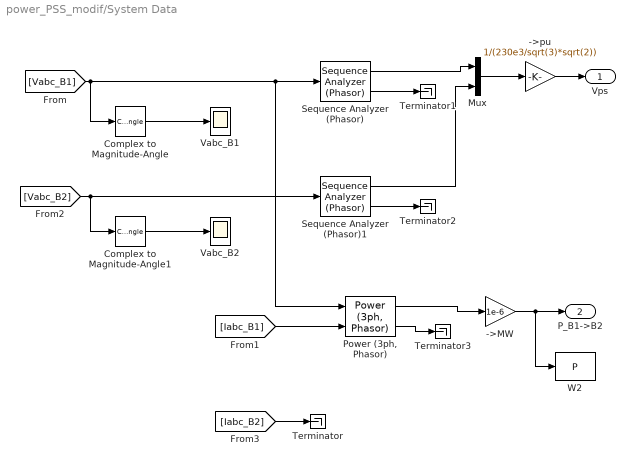
== system power_PSS_modif/System Data ==
  ->MW : Gain  Gain=1e-6  SaturateOnIntegerOverflow=on  OutDataTypeStr=Inherit: Same as input  ParamDataTypeStr=Inherit: Same as input
  ->pu : Gain  Gain=1/(230e3/sqrt(3)*sqrt(2))  SaturateOnIntegerOverflow=on  OutDataTypeStr=Inherit: Same as input  ParamDataTypeStr=Inherit: Same as input
  Complex to Magnitude-Angle : ComplexToMagnitudeAngle  Output=Magnitude
  Complex to Magnitude-Angle1 : ComplexToMagnitudeAngle  Output=Magnitude
  Mux : Mux  Inputs=2
  "Power (3ph, Phasor)" : spsPower3phPhasorLib/Power (3ph, Phasor)
      settings: SourceProductBaseCode=PS
  Sequence Analyzer (Phasor) : spsSequenceAnalyzerPhasorLib/Sequence Analyzer (Phasor)  seq=Positive
      settings: SourceProductBaseCode=PS
  Sequence Analyzer (Phasor)1 : spsSequenceAnalyzerPhasorLib/Sequence Analyzer (Phasor)  seq=Positive
      settings: SourceProductBaseCode=PS
  Terminator{,1..3} (4 alike) : Terminator
  Vabc_B1 : Scope
  Vabc_B2 : Scope
  W2 : ToWorkspace  VariableName=P  SampleTime=1/60
  Vps : Outport  VectorParamsAs1DForOutWhenUnconnected=off
  P_B1->B2 : Outport  Port=2  VectorParamsAs1DForOutWhenUnconnected=off
  wires:
  [Vabc_B1] -> Sequence Analyzer (Phasor)/1, "Power (3ph, Phasor)"/1, Complex to Magnitude-Angle/1
  [Vabc_B2] -> Sequence Analyzer (Phasor)1/1, Complex to Magnitude-Angle1/1
  [Iabc_B2] -> Terminator/1
  Sequence Analyzer (Phasor)/2 -> Terminator1/1
  Sequence Analyzer (Phasor)1/2 -> Terminator2/1
  Sequence Analyzer (Phasor)1/1 -> Mux/2
  [Iabc_B1] -> "Power (3ph, Phasor)"/2
  ->pu/1 -> Vps/1
  Sequence Analyzer (Phasor)/1 -> Mux/1
  Mux/1 -> ->pu/1
  ->MW/1 -> P_B1->B2/1, W2/1
  Complex to Magnitude-Angle/1 -> Vabc_B1/1
  Complex to Magnitude-Angle1/1 -> Vabc_B2/1
  "Power (3ph, Phasor)"/1 -> ->MW/1
  "Power (3ph, Phasor)"/2 -> Terminator3/1

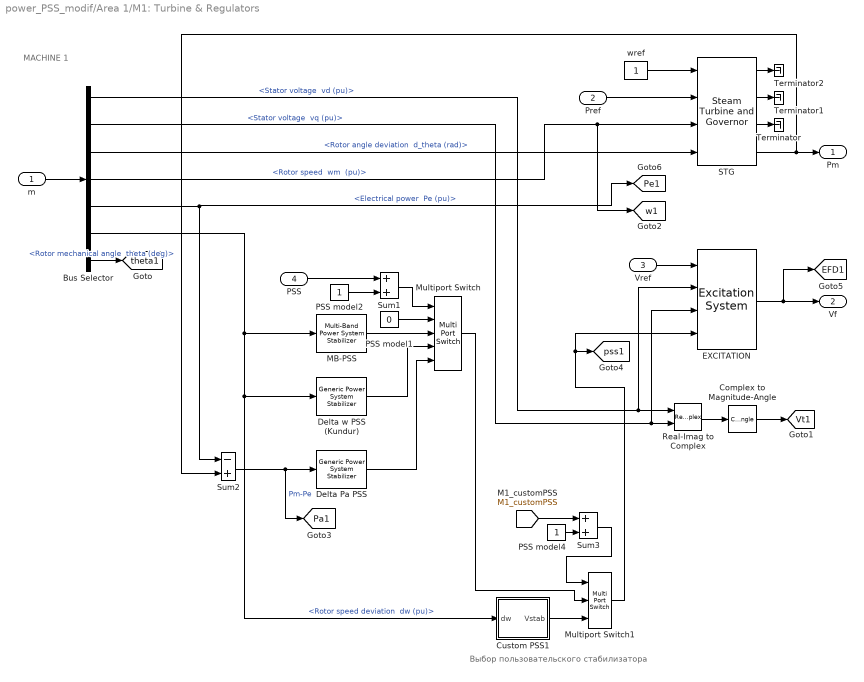
== system power_PSS_modif/Area 1/M1: Turbine & Regulators ==
  note: Выбор пользовательского стабилизатора
  note: MACHINE 1
  m : Inport
  Pref : Inport  Port=2
  Vref : Inport  Port=3
  PSS : Inport  Port=4
  Bus Selector : BusSelector  OutputSignals="dq0 components.Stator voltage  vd (pu),dq0 components.Stator voltage  vq (pu),Mechanical.Rotor angle deviation  d_theta (rad),Mechanical.Rotor speed  wm  (pu),Mechanical.Electrical power  Pe (pu),Mechanical.Rotor speed deviation  dw (pu),Mechanical.Rotor mechanical angle  theta (deg)"
  Complex to Magnitude-Angle : ComplexToMagnitudeAngle  Output=Magnitude
  Custom PSS1 : Subsystem  mask{limits=[-1 1]}
      mask prompts: limits "Limits [lower upper]"
      mask init:
      | lower = limits(1);
      | upper = limits(2);
  "Delta Pa PSS " : spsGenericPowerSystemStabilizerLib/Generic Power System Stabilizer  Tsensor=15e-3  K=2.5*1.25  Twashout=1  Tleadlag1=[60e-3 1]  Tleadlag2=[0 0]  VSlimits=[-0.15 0.15]  Vinit=0  Plot_On=off  MagdB_On=off  FreqRange=logspace(-2,2,500)
      settings: SourceProductBaseCode=PS
  "Delta w PSS (Kundur) " : spsGenericPowerSystemStabilizerLib/Generic Power System Stabilizer  Tsensor=15e-3  K=30  Twashout=10  Tleadlag1=[50e-3 20e-3]  Tleadlag2=[3 5.4]  VSlimits=[-0.15 0.15]  Vinit=0  Plot_On=off  MagdB_On=off  FreqRange=logspace(-2,2,500)
      settings: SourceProductBaseCode=PS
  EXCITATION : spsExcitationSystemLib/Excitation System  tr=20e-3  reg=[ 200, 0.001 ]  exc=[ 1, 0 ]  tgr=[ 0, 0 ]  damp=[ 0, 0 ]  sat=[ 0, 0 ]  lim=[ 0 , 12.3, 0 ]  v0=[1 1.7067]
      settings: SourceProductBaseCode=PS
  "MB-PSS " : spsMultiBandPowerSystemStabilizerLib/Multi-Band Power System Stabilizer  OperationMode=Simplified settings  Kg=1.0  GL=[0.2 30]  GI=[1.25 40]  GH=[12.0 160]  GLd=[66 66 9.4]  TcLF=[1.667 2 0 0 0 0 2 2.4 0 0 0 0 1 1]  GId=[66 66 47.6]  TcIF=[1 1 0.25 0.3 0 0 1 1 0.3 0.36 0 0 0 0]  GHd=[66 66 233]  TcHF="[0.01 0.012 0 0 0 0  0.012 0.0144 0 0 0 0 1 1]"  LIM=[.075 .15 .15 .15]  Plot_On=off  MagdB_On=off  FreqRange=logspace(-2,2,500)
      settings: SourceProductBaseCode=PS
  Multiport Switch : MultiPortSwitch  Inputs=4  InputSameDT=on
  Multiport Switch1 : MultiPortSwitch  Inputs=2  InputSameDT=on
  PSS model1 : Constant  Value=0
  PSS model2 : Constant
  PSS model4 : Constant
  Real-Imag to Complex : RealImagToComplex
  STG : spsSteamTurbineandGovernorLib/Steam Turbine and Governor  gentype=Tandem-compound (single mass)  reg1="[ 1  0.05    0 ]"  reg2="[ 0.001  0.15 ]"  reg3="[ -0.1  0.1  0  4.496 ]"  N=3600  turb1="[ 0  10   3.3   0.5   ]"  turb2="[   0   0.36    0.36   0.28   ]"  HA="[ 0.046  1.430  1.465   0.192 ]"  KA="[ 90.44  53.88  64.59   62.94  ]"  DA="[ 0.0115  0.3575  0.3663   0.0137  ]"  ini1=0.73731  ini2=[0.779316,-31.4247]
      settings: SourceProductBaseCode=PS
  Sum1 : Sum  InputSameDT=on  SaturateOnIntegerOverflow=on  OutDataTypeStr=Inherit: Same as first input
  Sum2 : Sum  Inputs=-+  InputSameDT=on  SaturateOnIntegerOverflow=on  OutDataTypeStr=Inherit: Same as first input
  Sum3 : Sum  InputSameDT=on  SaturateOnIntegerOverflow=on  OutDataTypeStr=Inherit: Same as first input
  Terminator : Terminator
  Terminator1 : Terminator
  Terminator2 : Terminator
  wref : Constant
  Pm : Outport  InitialOutput=0  VectorParamsAs1DForOutWhenUnconnected=off
  Vf : Outport  Port=2  InitialOutput=0  VectorParamsAs1DForOutWhenUnconnected=off
  tag scope: EFD1=global, Pa1=global, Pe1=global, Vt1=global, pss1=global, theta1=global, w1=global
  wires:
  Bus Selector/1 -> Real-Imag to Complex/1, EXCITATION/2  "<Stator voltage  vd (pu)>"
  Bus Selector/2 -> Real-Imag to Complex/2, EXCITATION/3  "<Stator voltage  vq (pu)>"
  wref/1 -> STG/1
  Pref/1 -> STG/2
  m/1 -> Bus Selector/1
  Vref/1 -> EXCITATION/1
  Real-Imag to Complex/1 -> Complex to Magnitude-Angle/1
  EXCITATION/1 -> Vf/1, [EFD1]
  Complex to Magnitude-Angle/1 -> [Vt1]
  Bus Selector/7 -> [theta1]  "<Rotor mechanical angle  theta (deg)>"
  PSS model1/1 -> Multiport Switch/2
  "MB-PSS "/1 -> Multiport Switch/3
  "Delta w PSS (Kundur) "/1 -> Multiport Switch/4
  "Delta Pa PSS "/1 -> Multiport Switch/5
  PSS model2/1 -> Sum1/2
  Sum1/1 -> Multiport Switch/1
  PSS/1 -> Sum1/1
  Bus Selector/4 -> [w1], STG/3  "<Rotor speed  wm  (pu)>"
  Bus Selector/5 -> [Pe1], Sum2/1  "<Electrical power  Pe (pu)>"
  Bus Selector/6 -> Custom PSS1/1(dw), "Delta w PSS (Kundur) "/1, "MB-PSS "/1  "<Rotor speed deviation  dw (pu)>"
  Sum2/1 -> [Pa1], "Delta Pa PSS "/1  "Pm-Pe"
  STG/3 -> Terminator/1
  STG/4 -> Pm/1, Sum2/2
  STG/2 -> Terminator1/1
  STG/1 -> Terminator2/1
  Bus Selector/3 -> STG/4  "<Rotor angle deviation  d_theta (rad)>"
  Sum3/1 -> Multiport Switch1/1
  PSS model4/1 -> Sum3/2
  Multiport Switch1/1 -> [pss1], EXCITATION/4
  Multiport Switch/1 -> Multiport Switch1/2
  [M1_customPSS] -> Sum3/1
  Custom PSS1/1(Vstab) -> Multiport Switch1/3

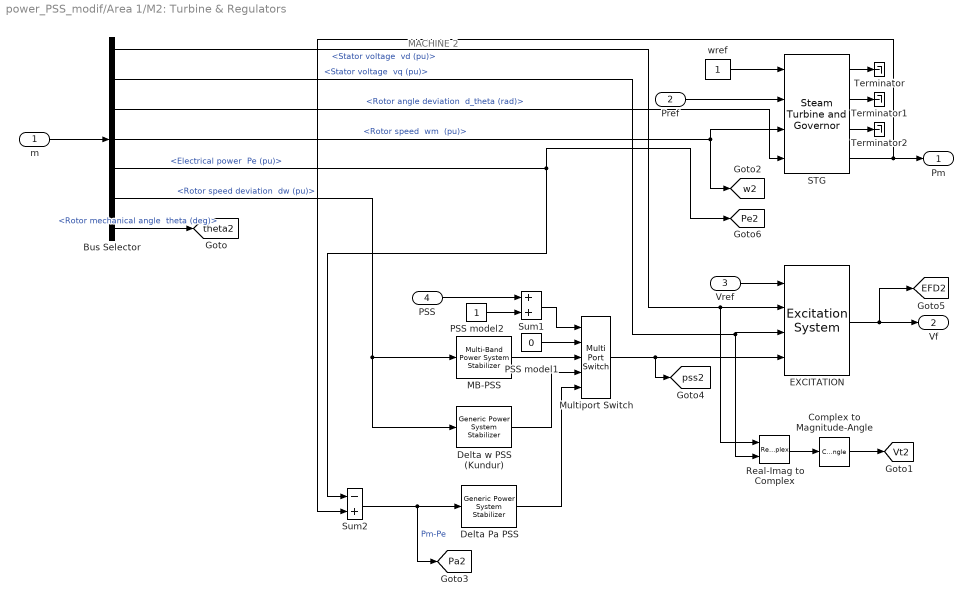
== system power_PSS_modif/Area 1/M2: Turbine & Regulators ==
  note: MACHINE 2
  m : Inport
  Pref : Inport  Port=2
  Vref : Inport  Port=3
  PSS : Inport  Port=4
  Bus Selector : BusSelector  OutputSignals="dq0 components.Stator voltage  vd (pu),dq0 components.Stator voltage  vq (pu),Mechanical.Rotor angle deviation  d_theta (rad),Mechanical.Rotor speed  wm  (pu),Mechanical.Electrical power  Pe (pu),Mechanical.Rotor speed deviation  dw (pu),Mechanical.Rotor mechanical angle  theta (deg)"
  Complex to Magnitude-Angle : ComplexToMagnitudeAngle  Output=Magnitude
  "Delta Pa PSS " : spsGenericPowerSystemStabilizerLib/Generic Power System Stabilizer  Tsensor=15e-3  K=2.5*1.25  Twashout=1  Tleadlag1=[60e-3 1]  Tleadlag2=[0 0]  VSlimits=[-0.15 0.15]  Vinit=0  Plot_On=off  MagdB_On=on  FreqRange=logspace(-2,2,500)
      settings: SourceProductBaseCode=PS
  "Delta w PSS (Kundur) " : spsGenericPowerSystemStabilizerLib/Generic Power System Stabilizer  Tsensor=15e-3  K=30  Twashout=10  Tleadlag1=[50e-3 20e-3]  Tleadlag2=[3 5.4]  VSlimits=[-0.15 0.15]  Vinit=0  Plot_On=off  MagdB_On=on  FreqRange=logspace(-2,2,500)
      settings: SourceProductBaseCode=PS
  EXCITATION : spsExcitationSystemLib/Excitation System  tr=20e-3  reg=[ 200, 0.001 ]  exc=[ 1, 0 ]  tgr=[ 0, 0 ]  damp=[ 0, 0 ]  sat=[ 0, 0 ]  lim=[ 0 , 12.3, 0 ]  v0=[1 1.4501]
      settings: SourceProductBaseCode=PS
  "MB-PSS " : spsMultiBandPowerSystemStabilizerLib/Multi-Band Power System Stabilizer  OperationMode=Simplified settings  Kg=1.0  GL=[0.2 30]  GI=[1.25 40]  GH=[12.0 160]  GLd=[66 66 9.4]  TcLF=[1.667 2 0 0 0 0 2 2.4 0 0 0 0 1 1]  GId=[66 66 47.6]  TcIF=[1 1 0.25 0.3 0 0 1 1 0.3 0.36 0 0 0 0]  GHd=[66 66 233]  TcHF="[0.01 0.012 0 0 0 0  0.012 0.0144 0 0 0 0 1 1]"  LIM=[.075 .15 .15 .15]  Plot_On=off  MagdB_On=off  FreqRange=logspace(-2,2,500)
      settings: SourceProductBaseCode=PS
  Multiport Switch : MultiPortSwitch  Inputs=4  InputSameDT=on
  PSS model1 : Constant  Value=0
  PSS model2 : Constant
  Real-Imag to Complex : RealImagToComplex
  STG : spsSteamTurbineandGovernorLib/Steam Turbine and Governor  gentype=Tandem-compound (single mass)  reg1="[ 1  0.05    0 ]"  reg2="[ 0.001  0.15 ]"  reg3="[ -0.1  0.1  0  4.496 ]"  N=3600  turb1="[ 0  10   3.3   0.5   ]"  turb2="[   0   0.36    0.36   0.28   ]"  HA="[ 0.046  1.430  1.465   0.192 ]"  KA="[ 90.44  53.88  64.59   62.94  ]"  DA="[ 0.0115  0.3575  0.3663   0.0137  ]"  ini1=0.5951  ini2=[0.779243,-42.8075]
      settings: SourceProductBaseCode=PS
  Sum1 : Sum  InputSameDT=on  SaturateOnIntegerOverflow=on  OutDataTypeStr=Inherit: Same as first input
  Sum2 : Sum  Inputs=-+  InputSameDT=on  SaturateOnIntegerOverflow=on  OutDataTypeStr=Inherit: Same as first input
  Terminator : Terminator
  Terminator1 : Terminator
  Terminator2 : Terminator
  wref : Constant
  Pm : Outport  InitialOutput=0  VectorParamsAs1DForOutWhenUnconnected=off
  Vf : Outport  Port=2  InitialOutput=0  VectorParamsAs1DForOutWhenUnconnected=off
  tag scope: EFD2=global, Pa2=global, Pe2=global, Vt2=global, pss2=global, theta2=global, w2=global
  wires:
  Sum2/1 -> [Pa2], "Delta Pa PSS "/1  "Pm-Pe"
  Bus Selector/6 -> "MB-PSS "/1, "Delta w PSS (Kundur) "/1  "<Rotor speed deviation  dw (pu)>"
  Bus Selector/5 -> [Pe2], Sum2/1  "<Electrical power  Pe (pu)>"
  Bus Selector/4 -> STG/3, [w2]  "<Rotor speed  wm  (pu)>"
  PSS/1 -> Sum1/1
  Sum1/1 -> Multiport Switch/1
  PSS model2/1 -> Sum1/2
  "Delta Pa PSS "/1 -> Multiport Switch/5
  "Delta w PSS (Kundur) "/1 -> Multiport Switch/4
  "MB-PSS "/1 -> Multiport Switch/3
  PSS model1/1 -> Multiport Switch/2
  Multiport Switch/1 -> [pss2], EXCITATION/4
  Bus Selector/7 -> [theta2]  "<Rotor mechanical angle  theta (deg)>"
  Complex to Magnitude-Angle/1 -> [Vt2]
  EXCITATION/1 -> [EFD2], Vf/1
  Real-Imag to Complex/1 -> Complex to Magnitude-Angle/1
  Vref/1 -> EXCITATION/1
  Pref/1 -> STG/2
  wref/1 -> STG/1
  Bus Selector/2 -> Real-Imag to Complex/2, EXCITATION/3  "<Stator voltage  vq (pu)>"
  Bus Selector/1 -> Real-Imag to Complex/1, EXCITATION/2  "<Stator voltage  vd (pu)>"
  STG/1 -> Terminator/1
  STG/2 -> Terminator1/1
  STG/3 -> Terminator2/1
  STG/4 -> Pm/1, Sum2/2
  Bus Selector/3 -> STG/4  "<Rotor angle deviation  d_theta (rad)>"
  m/1 -> Bus Selector/1
